simulink model "torque_control_simulation_sm"  (R2023b)
settings: Solver=VariableStepAuto  StartTime=0.0  StopTime=10.0  RelTol=1e-3
undefined symbols (not defined in the file): G_v, k_t, L_a, R_a
libraries: cstblocks x2
settings Model: Creator=adamo  LastModifiedBy=adamo

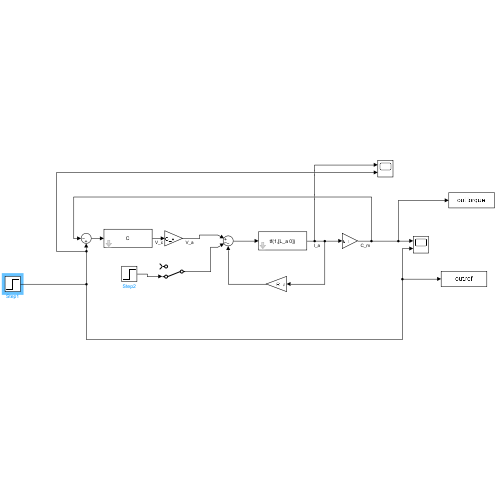
[thumbnail: Simulink's stored preview of the top-level diagram]
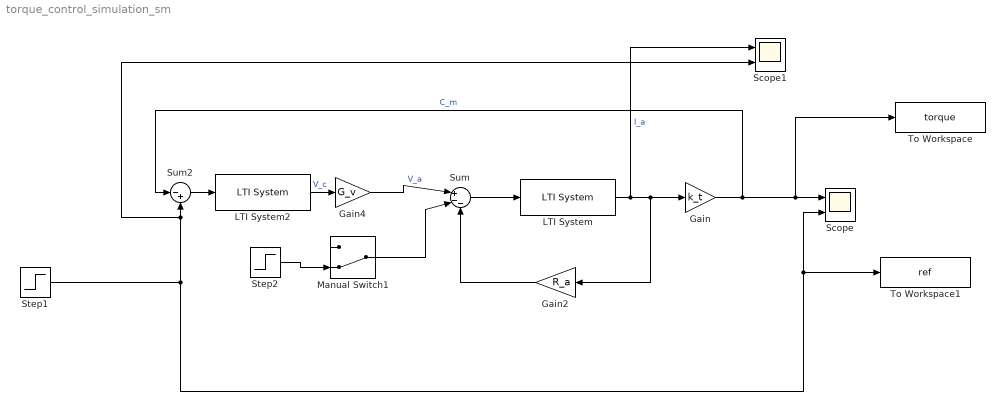
== system torque_control_simulation_sm ==
  Gain : Gain  Gain=k_t
  Gain2 : Gain  Gain=R_a
  Gain4 : Gain  Gain=G_v
  LTI System : cstblocks/LTI System  sys=tf(1,[L_a 0])  IC=[]  PadeOrder=0
  LTI System2 : cstblocks/LTI System  sys=C  IC=[]  PadeOrder=0
  Manual Switch1 : ManualSwitch  CurrentSetting=0
  Scope : Scope  NumInputPorts=2
  Scope1 : Scope  NumInputPorts=2
  Step1 : Step  Time=0  SampleTime=0
  Step2 : Step  Time=5  SampleTime=0
  Sum : Sum  Inputs=|+--
  Sum2 : Sum  Inputs=|-+
  To Workspace : ToWorkspace  VariableName=torque  SaveFormat=Timeseries  SampleTime=-1
  To Workspace1 : ToWorkspace  VariableName=ref  SaveFormat=Timeseries  SampleTime=-1
  wires:
  Sum/1 -> LTI System/1
  LTI System/1 -> Gain2/1, Gain/1, Scope1/1  "I_a"
  Gain2/1 -> Sum/3
  Gain4/1 -> Sum/1  "V_a"
  LTI System2/1 -> Gain4/1  "V_c"
  Sum2/1 -> LTI System2/1
  Step1/1 -> To Workspace1/1, Scope/2, Scope1/2, Sum2/2
  Step2/1 -> Manual Switch1/2
  Manual Switch1/1 -> Sum/2
  Gain/1 -> Sum2/1, To Workspace/1, Scope/1  "C_m"
